simulink model "compare"  (R2016a)
settings: Solver=VariableStepAuto  StartTime=0.0  StopTime=200  RelTol=1e-3
settings Model: Creator=ASUS  LastModifiedBy=ASUS

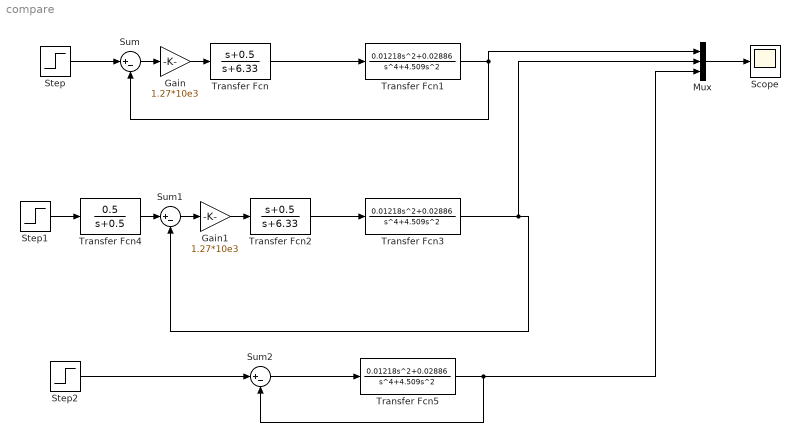
== system compare ==
  Gain : Gain  Gain=1.27*10e3
  Gain1 : Gain  Gain=1.27*10e3
  Mux : Mux  Inputs=3
  Scope : Scope
  Step : Step  SampleTime=0
  Step1 : Step  SampleTime=0
  Step2 : Step  SampleTime=0
  Sum : Sum  Inputs=|+-
  Sum1 : Sum  Inputs=|+-
  Sum2 : Sum  Inputs=|+-
  Transfer Fcn : TransferFcn  Numerator=[1 0.5]  Denominator=[1 6.33]
  Transfer Fcn1 : TransferFcn  Numerator=[0.01218 0 0.02886]  Denominator="[1 0  4.509 0 0 ]"
  Transfer Fcn2 : TransferFcn  Numerator=[1 0.5]  Denominator=[1 6.33]
  Transfer Fcn3 : TransferFcn  Numerator=[0.01218 0 0.02886]  Denominator="[1 0  4.509 0 0 ]"
  Transfer Fcn4 : TransferFcn  Numerator=[0.5]  Denominator=[1 0.5]
  Transfer Fcn5 : TransferFcn  Numerator=[0.01218 0 0.02886]  Denominator="[1 0  4.509 0 0 ]"
  wires:
  Step/1 -> Sum/1
  Transfer Fcn/1 -> Transfer Fcn1/1
  Sum/1 -> Gain/1
  Gain/1 -> Transfer Fcn/1
  Transfer Fcn1/1 -> Sum/2, Mux/1
  Transfer Fcn4/1 -> Sum1/1
  Transfer Fcn2/1 -> Transfer Fcn3/1
  Step1/1 -> Transfer Fcn4/1
  Sum1/1 -> Gain1/1
  Gain1/1 -> Transfer Fcn2/1
  Transfer Fcn3/1 -> Mux/2, Sum1/2
  Step2/1 -> Sum2/1
  Transfer Fcn5/1 -> Mux/3, Sum2/2
  Sum2/1 -> Transfer Fcn5/1
  Mux/1 -> Scope/1
